simulink model "PruebaFinal"  (R2025b)
settings: Solver=VariableStepAuto  StartTime=0.0  StopTime=inf  RelTol=1e-3
libraries: Drive_Mode_Librery x1, Gear_Selection_Library x1, Hydraulic_Pressure_Control_Library x1, TCC_Control_Library x1

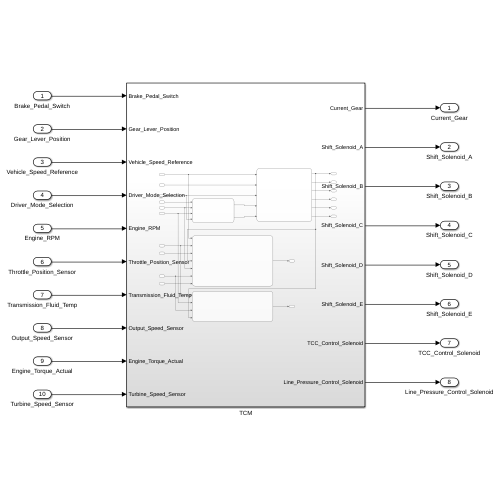
[thumbnail: Simulink's stored preview of the top-level diagram]
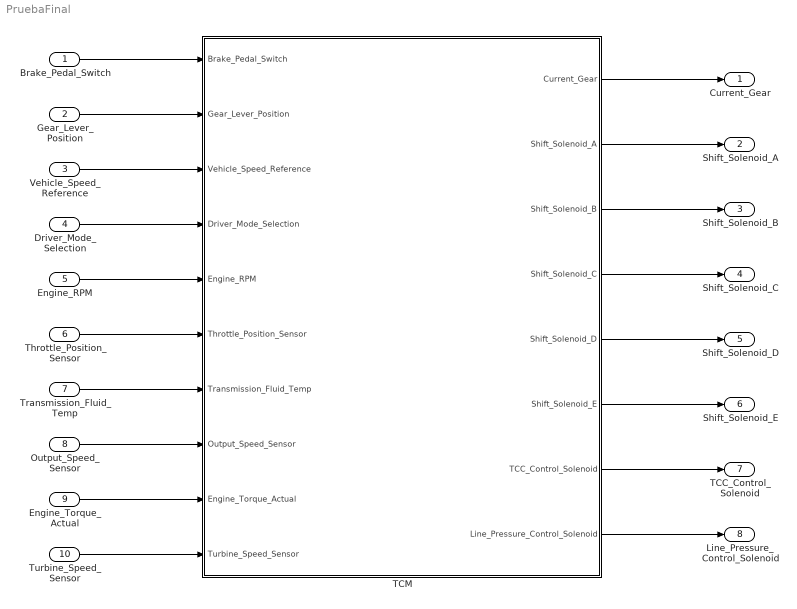
== system PruebaFinal ==
  Brake_Pedal_Switch : Inport  OutDataTypeStr=uint8  PortDimensions=1
  Gear_Lever_Position : Inport  Port=2  OutDataTypeStr=uint8  PortDimensions=1
  Vehicle_Speed_Reference : Inport  Port=3  OutDataTypeStr=uint8  PortDimensions=1
  Driver_Mode_Selection : Inport  Port=4  OutDataTypeStr=uint8  PortDimensions=1
  Engine_RPM : Inport  Port=5  OutDataTypeStr=uint16  PortDimensions=1
  Throttle_Position_Sensor : Inport  Port=6  OutDataTypeStr=uint8  PortDimensions=1
  Transmission_Fluid_Temp : Inport  Port=7  OutDataTypeStr=int8  PortDimensions=1
  Output_Speed_Sensor : Inport  Port=8  OutDataTypeStr=uint16  PortDimensions=1
  Engine_Torque_Actual : Inport  Port=9  OutDataTypeStr=int16  PortDimensions=1
  Turbine_Speed_Sensor : Inport  Port=10  OutDataTypeStr=uint16  PortDimensions=1
  TCM : Subsystem
  Current_Gear : Outport  OutDataTypeStr=uint8  PortDimensions=1
  Shift_Solenoid_A : Outport  Port=2  OutDataTypeStr=uint8  PortDimensions=1
  Shift_Solenoid_B : Outport  Port=3  OutDataTypeStr=uint8  PortDimensions=1
  Shift_Solenoid_C : Outport  Port=4  OutDataTypeStr=uint8  PortDimensions=1
  Shift_Solenoid_D : Outport  Port=5  OutDataTypeStr=uint8  PortDimensions=1
  Shift_Solenoid_E : Outport  Port=6  OutDataTypeStr=uint8  PortDimensions=1
  TCC_Control_Solenoid : Outport  Port=7  OutDataTypeStr=uint8  PortDimensions=1
  Line_Pressure_Control_Solenoid : Outport  Port=8  OutDataTypeStr=uint8  PortDimensions=1
  wires:
  TCM/1(Current_Gear) -> Current_Gear/1
  TCM/2(Shift_Solenoid_A) -> Shift_Solenoid_A/1
  TCM/3(Shift_Solenoid_B) -> Shift_Solenoid_B/1
  TCM/4(Shift_Solenoid_C) -> Shift_Solenoid_C/1
  TCM/5(Shift_Solenoid_D) -> Shift_Solenoid_D/1
  TCM/6(Shift_Solenoid_E) -> Shift_Solenoid_E/1
  TCM/7(TCC_Control_Solenoid) -> TCC_Control_Solenoid/1
  TCM/8(Line_Pressure_Control_Solenoid) -> Line_Pressure_Control_Solenoid/1
  Brake_Pedal_Switch/1 -> TCM/1(Brake_Pedal_Switch)
  Gear_Lever_Position/1 -> TCM/2(Gear_Lever_Position)
  Vehicle_Speed_Reference/1 -> TCM/3(Vehicle_Speed_Reference)
  Driver_Mode_Selection/1 -> TCM/4(Driver_Mode_Selection)
  Engine_RPM/1 -> TCM/5(Engine_RPM)
  Throttle_Position_Sensor/1 -> TCM/6(Throttle_Position_Sensor)
  Transmission_Fluid_Temp/1 -> TCM/7(Transmission_Fluid_Temp)
  Output_Speed_Sensor/1 -> TCM/8(Output_Speed_Sensor)
  Engine_Torque_Actual/1 -> TCM/9(Engine_Torque_Actual)
  Turbine_Speed_Sensor/1 -> TCM/10(Turbine_Speed_Sensor)

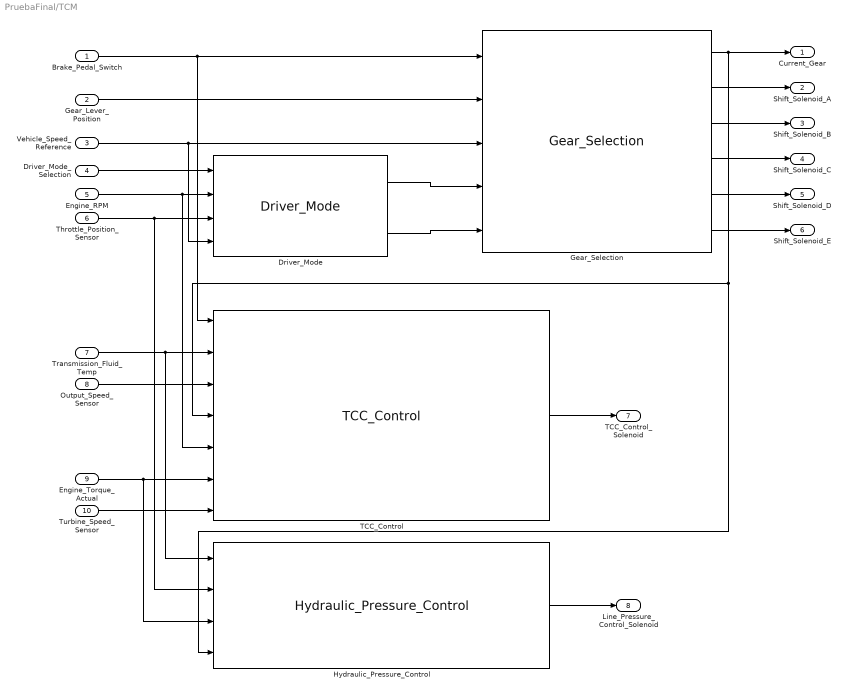
== system PruebaFinal/TCM ==
  Brake_Pedal_Switch : Inport  OutDataTypeStr=uint8  PortDimensions=1
  Gear_Lever_Position : Inport  Port=2  OutDataTypeStr=uint8  PortDimensions=1
  Vehicle_Speed_Reference : Inport  Port=3  OutDataTypeStr=uint8  PortDimensions=1
  Driver_Mode_Selection : Inport  Port=4  OutDataTypeStr=uint8  PortDimensions=1
  Engine_RPM : Inport  Port=5  OutDataTypeStr=uint16  PortDimensions=1
  Throttle_Position_Sensor : Inport  Port=6  OutDataTypeStr=uint8  PortDimensions=1
  Transmission_Fluid_Temp : Inport  Port=7  OutDataTypeStr=int8  PortDimensions=1
  Output_Speed_Sensor : Inport  Port=8  OutDataTypeStr=uint16  PortDimensions=1
  Engine_Torque_Actual : Inport  Port=9  OutDataTypeStr=int16  PortDimensions=1
  Turbine_Speed_Sensor : Inport  Port=10  OutDataTypeStr=uint16  PortDimensions=1
  Driver_Mode : Drive_Mode_Librery/Driver_Mode  SystemSampleTime=-1  VariantActivationTime=update diagram  EmptyChoice=off  PassThrough=off  PassThroughVariantControl=(default)  EmptyChoiceVariantControl=(default)  AllowFlexibleInterface=on  Latency=0  AutoFrameSizeCalculation=off
  Gear_Selection : Gear_Selection_Library/Gear_Selection  SystemSampleTime=-1  VariantActivationTime=update diagram  EmptyChoice=off  PassThrough=off  PassThroughVariantControl=(default)  EmptyChoiceVariantControl=(default)  AllowFlexibleInterface=on  Latency=0  AutoFrameSizeCalculation=off
  Hydraulic_Pressure_Control : Hydraulic_Pressure_Control_Library/Hydraulic_Pressure_Control  SystemSampleTime=-1  VariantActivationTime=update diagram  EmptyChoice=off  PassThrough=off  PassThroughVariantControl=(default)  EmptyChoiceVariantControl=(default)  AllowFlexibleInterface=on  Latency=0  AutoFrameSizeCalculation=off
  TCC_Control : TCC_Control_Library/TCC_Control  SystemSampleTime=-1  VariantActivationTime=update diagram  EmptyChoice=off  PassThrough=off  PassThroughVariantControl=(default)  EmptyChoiceVariantControl=(default)  AllowFlexibleInterface=on  Latency=0  AutoFrameSizeCalculation=off
      link override SlipMode_F/2-D Lookup Table: BreakpointsForDimension1DataTypeStr=uint8  BreakpointsForDimension2DataTypeStr=int16  ExtrapMethod=Clip
  Current_Gear : Outport  OutDataTypeStr=uint8  PortDimensions=1
  Shift_Solenoid_A : Outport  Port=2  OutDataTypeStr=uint8  PortDimensions=1
  Shift_Solenoid_B : Outport  Port=3  OutDataTypeStr=uint8  PortDimensions=1
  Shift_Solenoid_C : Outport  Port=4  OutDataTypeStr=uint8  PortDimensions=1
  Shift_Solenoid_D : Outport  Port=5  OutDataTypeStr=uint8  PortDimensions=1
  Shift_Solenoid_E : Outport  Port=6  OutDataTypeStr=uint8  PortDimensions=1
  TCC_Control_Solenoid : Outport  Port=7  OutDataTypeStr=uint8  PortDimensions=1
  Line_Pressure_Control_Solenoid : Outport  Port=8  OutDataTypeStr=uint8  PortDimensions=1
  wires:
  Gear_Selection/1 -> Hydraulic_Pressure_Control/4, TCC_Control/4, Current_Gear/1
  Gear_Selection/6 -> Shift_Solenoid_E/1
  Throttle_Position_Sensor/1 -> Hydraulic_Pressure_Control/2, Driver_Mode/3
  Brake_Pedal_Switch/1 -> TCC_Control/1, Gear_Selection/1
  Engine_RPM/1 -> TCC_Control/5, Driver_Mode/2
  Gear_Selection/4 -> Shift_Solenoid_C/1
  Driver_Mode/1 -> Gear_Selection/4
  Gear_Selection/5 -> Shift_Solenoid_D/1
  Driver_Mode/2 -> Gear_Selection/5
  Vehicle_Speed_Reference/1 -> Driver_Mode/4, Gear_Selection/3
  Gear_Lever_Position/1 -> Gear_Selection/2
  Gear_Selection/2 -> Shift_Solenoid_A/1
  Driver_Mode_Selection/1 -> Driver_Mode/1
  Gear_Selection/3 -> Shift_Solenoid_B/1
  TCC_Control/1 -> TCC_Control_Solenoid/1
  Transmission_Fluid_Temp/1 -> Hydraulic_Pressure_Control/1, TCC_Control/2
  Output_Speed_Sensor/1 -> TCC_Control/3
  Engine_Torque_Actual/1 -> Hydraulic_Pressure_Control/3, TCC_Control/6
  Turbine_Speed_Sensor/1 -> TCC_Control/7
  Hydraulic_Pressure_Control/1 -> Line_Pressure_Control_Solenoid/1
